simulink model "test0"  (R2016a)
settings: Solver=ode23  StartTime=0.0  StopTime=20  RelTol=1e-10
settings Model: Creator=wojta  LastModifiedBy=wojta

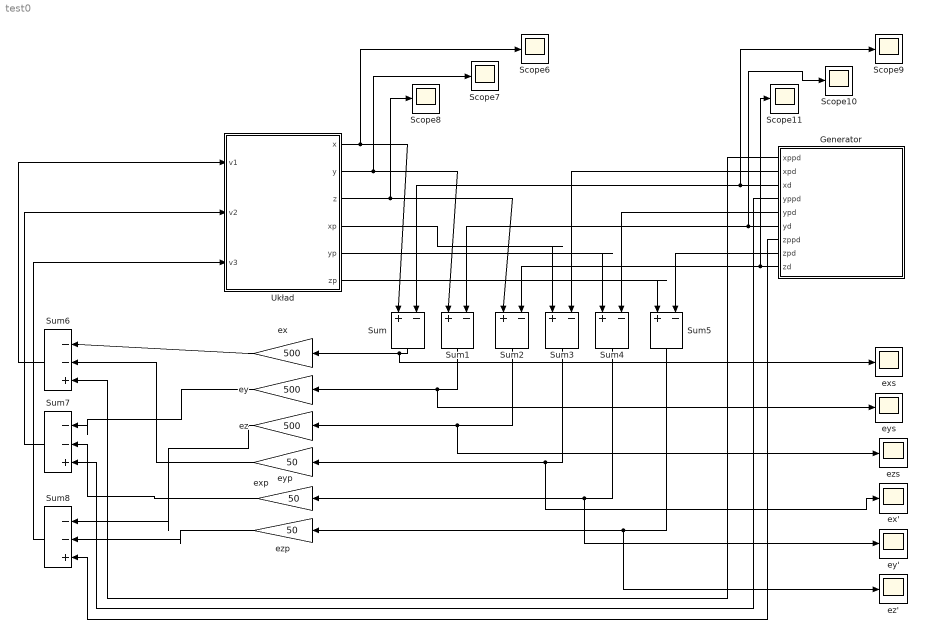
== system test0 ==
  Generator : Subsystem
  Scope{6..11} (6 alike) : Scope
  Sum{,1..5} (6 alike) : Sum  Inputs=|+-
  Sum6 : Sum  Inputs=|--+
  Sum7 : Sum  Inputs=|--+
  Sum8 : Sum  Inputs=|--+
  Układ : Subsystem
  ex : Gain  Gain=500
  ex' : Scope
  exp : Gain  Gain=50
  exs : Scope
  ey : Gain  Gain=500
  ey' : Scope
  eyp : Gain  Gain=50
  eys : Scope
  ez : Gain  Gain=500
  ez' : Scope
  ezp : Gain  Gain=50
  ezs : Scope
  wires:
  Układ/1(x) -> Scope6/1, Sum/1
  Generator/3(xd) -> Scope9/1, Sum/2
  Układ/2(y) -> Scope7/1, Sum1/1
  Generator/6(yd) -> Scope10/1, Sum1/2
  Układ/3(z) -> Scope8/1, Sum2/1
  Generator/9(zd) -> Scope11/1, Sum2/2
  Układ/4(xp) -> Sum3/1
  Generator/2(xpd) -> Sum3/2
  Układ/5(yp) -> Sum4/1
  Generator/5(ypd) -> Sum4/2
  Układ/6(zp) -> Sum5/1
  Generator/8(zpd) -> Sum5/2
  Sum/1 -> exs/1, ex/1
  Sum3/1 -> exp/1, ex'/1
  Sum4/1 -> ey'/1, eyp/1
  Sum5/1 -> ez'/1, ezp/1
  Sum2/1 -> ezs/1, ez/1
  Sum1/1 -> eys/1, ey/1
  ex/1 -> Sum6/1
  exp/1 -> Sum6/2
  Generator/1(xppd) -> Sum6/3
  Generator/4(yppd) -> Sum7/3
  Generator/7(zppd) -> Sum8/3
  ey/1 -> Sum7/1
  eyp/1 -> Sum7/2
  ezp/1 -> Sum8/2
  ez/1 -> Sum8/1
  Sum6/1 -> Układ/1(v1)
  Sum7/1 -> Układ/2(v2)
  Sum8/1 -> Układ/3(v3)

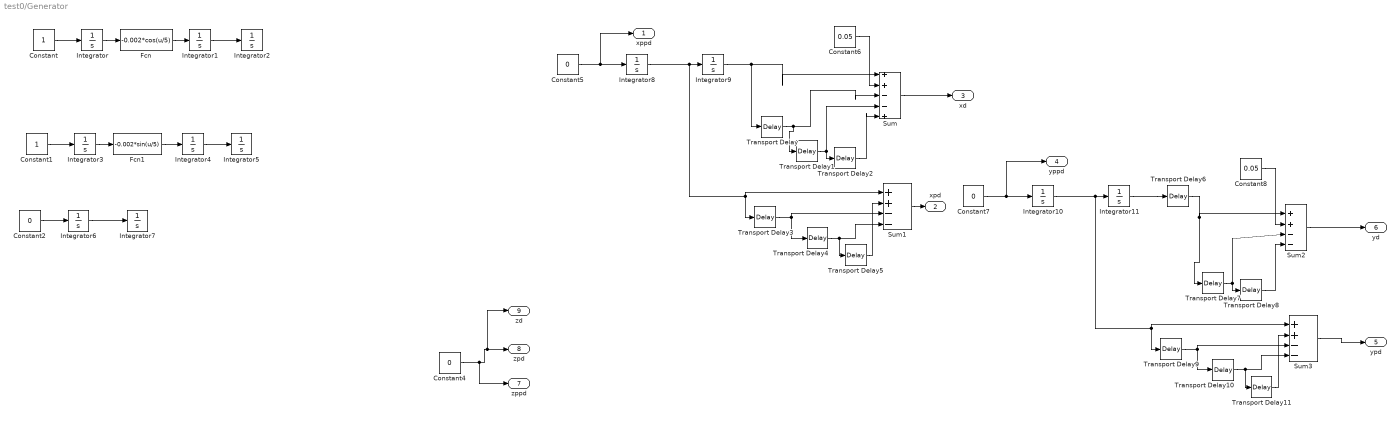
== system test0/Generator ==
  Constant : Constant
  Constant1 : Constant
  Constant{2,4..5,7} (4 alike) : Constant  Value=0
  Constant6 : Constant  Value=0.05
  Constant8 : Constant  Value=0.05
  Fcn : Fcn  Expr=-0.002*cos(u/5)
  Fcn1 : Fcn  Expr=-0.002*sin(u/5)
  Integrator{,1,3,5,7,9,11} (7 alike) : Integrator
  Integrator{4,6,8,10} (4 alike) : Integrator  InitialCondition=0.01
  Integrator2 : Integrator  InitialCondition=0.05
  Sum : Sum  Inputs=|++--+
  Sum1 : Sum  Inputs=|++--
  Sum2 : Sum  Inputs=|++--
  Sum3 : Sum  Inputs=|++--
  Transport Delay{,1..11} (12 alike) : TransportDelay  DelayTime=5
  xppd : Outport
  xpd : Outport  Port=2
  xd : Outport  Port=3
  yppd : Outport  Port=4
  ypd : Outport  Port=5
  yd : Outport  Port=6
  zppd : Outport  Port=7
  zpd : Outport  Port=8
  zd : Outport  Port=9
  wires:
  Constant/1 -> Integrator/1
  Integrator/1 -> Fcn/1
  Fcn/1 -> Integrator1/1
  Integrator1/1 -> Integrator2/1
  Constant1/1 -> Integrator3/1
  Integrator3/1 -> Fcn1/1
  Fcn1/1 -> Integrator4/1
  Integrator4/1 -> Integrator5/1
  Constant2/1 -> Integrator6/1
  Integrator6/1 -> Integrator7/1
  Constant4/1 -> zppd/1, zd/1, zpd/1
  Constant5/1 -> xppd/1, Integrator8/1
  Integrator8/1 -> Transport Delay3/1, Sum1/1, Integrator9/1
  Sum/1 -> xd/1
  Integrator9/1 -> Transport Delay/1, Sum/1
  Constant6/1 -> Sum/2
  Transport Delay/1 -> Transport Delay1/1, Sum/3
  Transport Delay1/1 -> Sum/4, Transport Delay2/1
  Transport Delay2/1 -> Sum/5
  Sum1/1 -> xpd/1
  Transport Delay3/1 -> Transport Delay4/1, Sum1/3
  Transport Delay4/1 -> Transport Delay5/1, Sum1/4
  Transport Delay5/1 -> Sum1/2
  Constant7/1 -> yppd/1, Integrator10/1
  Integrator10/1 -> Transport Delay9/1, Sum3/1, Integrator11/1
  Sum2/1 -> yd/1
  Integrator11/1 -> Transport Delay6/1
  Constant8/1 -> Sum2/2
  Transport Delay6/1 -> Sum2/1, Transport Delay7/1
  Transport Delay7/1 -> Sum2/3, Transport Delay8/1
  Transport Delay8/1 -> Sum2/4
  Transport Delay9/1 -> Transport Delay10/1, Sum3/3
  Transport Delay10/1 -> Transport Delay11/1, Sum3/4
  Transport Delay11/1 -> Sum3/2
  Sum3/1 -> ypd/1

== system test0/Układ ==
  v1 : Inport
  v2 : Inport  Port=2
  v3 : Inport  Port=3
  Constant3 : Constant  Value=1.6
  H : Subsystem
  O : Subsystem
  Obiekt : Subsystem
  Scope : Scope
  Scope1 : Scope
  Scope2 : Scope
  u : Subsystem
  x : Outport
  y : Outport  Port=2
  z : Outport  Port=3
  xp : Outport  Port=4
  yp : Outport  Port=5
  zp : Outport  Port=6
  wires:
  v3/1 -> u/3(v3)
  O/8(O32) -> u/14(O32)
  O/9(O33) -> u/15(O33)
  H/1(H1) -> u/4(H1)
  O/4(O21) -> u/10(O21)
  u/3(u3) -> Obiekt/3(u3)
  Obiekt/3(z) -> z/1, Scope2/1
  Obiekt/8(qp2) -> H/6(qp2)
  O/1(O11) -> u/7(O11)
  O/5(O22) -> u/11(O22)
  Obiekt/5(q2) -> H/3(q2), O/2(q2)
  Obiekt/7(qp3) -> H/7(qp3)
  H/3(H3) -> u/6(H3)
  H/2(H2) -> u/5(H2)
  Obiekt/4(q3) -> O/3(q3), H/4(q3)
  Obiekt/2(y) -> y/1, Scope1/1
  u/2(u2) -> Obiekt/2(u2)
  O/7(O31) -> u/13(O31)
  Obiekt/1(x) -> x/1, Scope/1
  Constant3/1 -> Obiekt/4(q4), O/4(q4), H/1(q4)
  Obiekt/9(qp1) -> H/5(qp1)
  O/2(O12) -> u/8(O12)
  u/1(u1) -> Obiekt/1(u1)
  O/3(O13) -> u/9(O13)
  Obiekt/6(q1) -> O/1(q1), H/2(q1)
  O/6(O23) -> u/12(O23)
  v1/1 -> u/1(v1)
  v2/1 -> u/2(v2)
  Obiekt/10(xp) -> xp/1
  Obiekt/11(yp) -> yp/1
  Obiekt/12(zp) -> zp/1

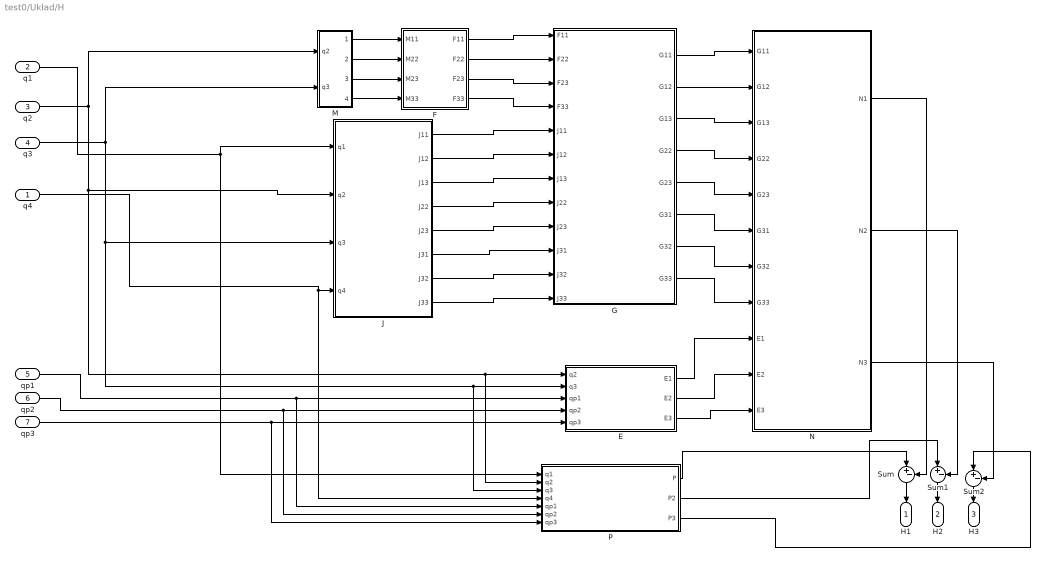
== system test0/Układ/H ==
  q4 : Inport
  q1 : Inport  Port=2
  q2 : Inport  Port=3
  q3 : Inport  Port=4
  qp1 : Inport  Port=5
  qp2 : Inport  Port=6
  qp3 : Inport  Port=7
  E : Subsystem
  F : Subsystem
  G : Subsystem
  J : Subsystem
  M : Subsystem
  N : Subsystem
  P : Subsystem
  Sum : Sum  Inputs=|+-
  Sum1 : Sum  Inputs=|+-
  Sum2 : Sum  Inputs=|+-
  H1 : Outport
  H2 : Outport  Port=2
  H3 : Outport  Port=3
  wires:
  q3/1 -> M/2(q3), P/3(q3), E/2(q3), J/3(q3)
  q1/1 -> P/1(q1), J/1(q1)
  q2/1 -> P/2(q2), E/1(q2), J/2(q2), M/1(q2)
  q4/1 -> P/4(q4), J/4(q4)
  F/1(F11) -> G/1(F11)
  F/2(F22) -> G/2(F22)
  F/3(F23) -> G/3(F23)
  F/4(F33) -> G/4(F33)
  J/1(J11) -> G/5(J11)
  J/2(J12) -> G/6(J12)
  J/3(J13) -> G/7(J13)
  J/4(J22) -> G/8(J22)
  J/5(J23) -> G/9(J23)
  J/6(J31) -> G/10(J31)
  J/7(J32) -> G/11(J32)
  J/8(J33) -> G/12(J33)
  qp1/1 -> P/5(qp1), E/3(qp1)
  qp2/1 -> P/6(qp2), E/4(qp2)
  qp3/1 -> P/7(qp3), E/5(qp3)
  E/3(E3) -> N/11(E3)
  E/2(E2) -> N/10(E2)
  E/1(E1) -> N/9(E1)
  G/8(G33) -> N/8(G33)
  G/7(G32) -> N/7(G32)
  G/6(G31) -> N/6(G31)
  G/5(G23) -> N/5(G23)
  G/4(G22) -> N/4(G22)
  G/2(G12) -> N/2(G12)
  G/3(G13) -> N/3(G13)
  G/1(G11) -> N/1(G11)
  Sum/1 -> H1/1
  Sum1/1 -> H2/1
  Sum2/1 -> H3/1
  N/1(N1) -> Sum/2
  N/2(N2) -> Sum1/2
  N/3(N3) -> Sum2/2
  P/1(P) -> Sum/1
  P/2(P2) -> Sum1/1
  P/3(P3) -> Sum2/1
  M/3(M23) -> F/3(M23)
  M/1(M11) -> F/1(M11)
  M/4("M33 ") -> F/4(M33)
  M/2(M22) -> F/2(M22)

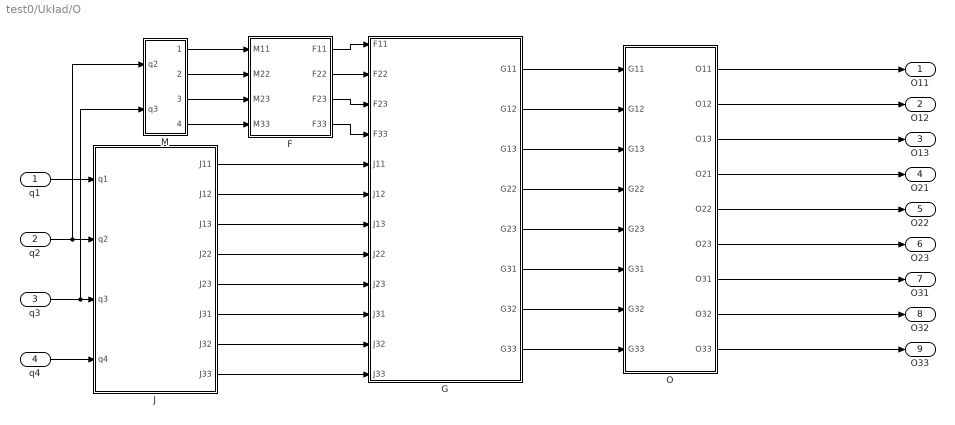
== system test0/Układ/O ==
  q1 : Inport
  q2 : Inport  Port=2
  q3 : Inport  Port=3
  q4 : Inport  Port=4
  F : Subsystem
  G : Subsystem
  J : Subsystem
  M : Subsystem
  O : Subsystem
  O11 : Outport
  O12 : Outport  Port=2
  O13 : Outport  Port=3
  O21 : Outport  Port=4
  O22 : Outport  Port=5
  O23 : Outport  Port=6
  O31 : Outport  Port=7
  O32 : Outport  Port=8
  O33 : Outport  Port=9
  wires:
  J/1(J11) -> G/5(J11)
  J/2(J12) -> G/6(J12)
  J/3(J13) -> G/7(J13)
  J/4(J22) -> G/8(J22)
  J/5(J23) -> G/9(J23)
  J/6(J31) -> G/10(J31)
  J/7(J32) -> G/11(J32)
  J/8(J33) -> G/12(J33)
  q3/1 -> J/3(q3), M/2(q3)
  q2/1 -> J/2(q2), M/1(q2)
  q1/1 -> J/1(q1)
  q4/1 -> J/4(q4)
  G/1(G11) -> O/1(G11)
  G/2(G12) -> O/2(G12)
  G/3(G13) -> O/3(G13)
  G/4(G22) -> O/4(G22)
  G/5(G23) -> O/5(G23)
  G/6(G31) -> O/6(G31)
  G/7(G32) -> O/7(G32)
  G/8(G33) -> O/8(G33)
  O/1(O11) -> O11/1
  O/2(O12) -> O12/1
  O/3(O13) -> O13/1
  O/4(O21) -> O21/1
  O/5(O22) -> O22/1
  O/6(O23) -> O23/1
  O/7(O31) -> O31/1
  O/8(O32) -> O32/1
  O/9(O33) -> O33/1
  M/3(M23) -> F/3(M23)
  M/1(M11) -> F/1(M11)
  M/4("M33 ") -> F/4(M33)
  M/2(M22) -> F/2(M22)
  F/1(F11) -> G/1(F11)
  F/2(F22) -> G/2(F22)
  F/3(F23) -> G/3(F23)
  F/4(F33) -> G/4(F33)

== system test0/Układ/Obiekt ==
  u1 : Inport
  u2 : Inport  Port=2
  u3 : Inport  Port=3
  q4 : Inport  Port=4
  Dynamika : Subsystem
  Kinematyka : Subsystem
  x : Outport
  y : Outport  Port=2
  z : Outport  Port=3
  q3 : Outport  Port=4
  q2 : Outport  Port=5
  q1 : Outport  Port=6
  qp3 : Outport  Port=7
  qp2 : Outport  Port=8
  qp1 : Outport  Port=9
  xp : Outport  Port=10
  yp : Outport  Port=11
  zp : Outport  Port=12
  wires:
  Dynamika/3(q3) -> q3/1, Kinematyka/3(q3)
  Dynamika/1(q1) -> q1/1, Kinematyka/1(q1)
  q4/1 -> Kinematyka/4(q4)
  Dynamika/2(q2) -> q2/1, Kinematyka/2(q2)
  Kinematyka/3(z) -> z/1
  Kinematyka/1(x) -> x/1
  Kinematyka/2(y) -> y/1
  u1/1 -> Dynamika/1(u1)
  u3/1 -> Dynamika/3(u3)
  u2/1 -> Dynamika/2(u2)
  Dynamika/4(qp3) -> Kinematyka/7(q3p), qp3/1
  Dynamika/6(qp1) -> Kinematyka/5(q1p), qp1/1
  Dynamika/5(qp2) -> Kinematyka/6(q2p), qp2/1
  Kinematyka/4(xp) -> xp/1
  Kinematyka/5(yp) -> yp/1
  Kinematyka/6(zp) -> zp/1

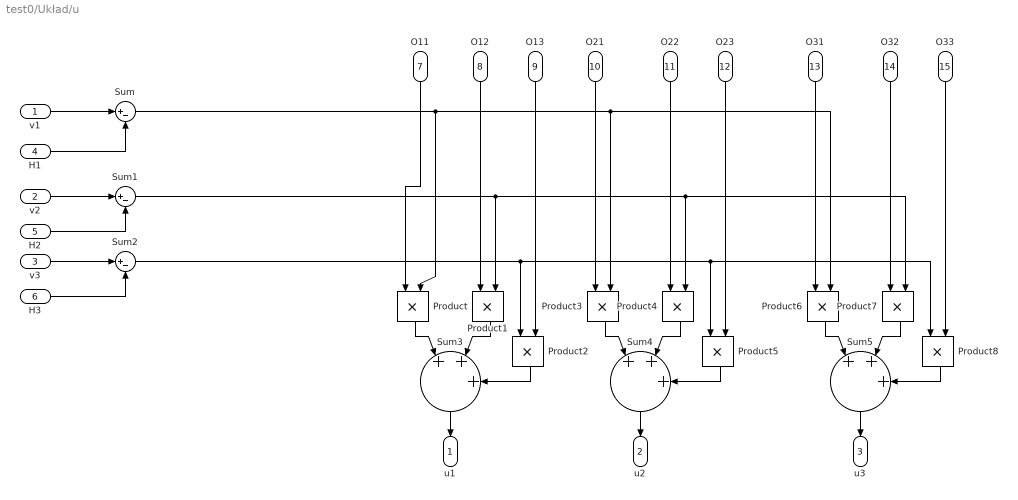
== system test0/Układ/u ==
  v1 : Inport
  v2 : Inport  Port=2
  v3 : Inport  Port=3
  H1 : Inport  Port=4
  H2 : Inport  Port=5
  H3 : Inport  Port=6
  O11 : Inport  Port=7
  O12 : Inport  Port=8
  O13 : Inport  Port=9
  O21 : Inport  Port=10
  O22 : Inport  Port=11
  O23 : Inport  Port=12
  O31 : Inport  Port=13
  O32 : Inport  Port=14
  O33 : Inport  Port=15
  Product{,1..8} (9 alike) : Product
  Sum : Sum  Inputs=|+-
  Sum1 : Sum  Inputs=|+-
  Sum2 : Sum  Inputs=|+-
  Sum3 : Sum  Inputs=|+++
  Sum4 : Sum  Inputs=|+++
  Sum5 : Sum  Inputs=|+++
  u1 : Outport
  u2 : Outport  Port=2
  u3 : Outport  Port=3
  wires:
  v1/1 -> Sum/1
  H1/1 -> Sum/2
  v2/1 -> Sum1/1
  H2/1 -> Sum1/2
  v3/1 -> Sum2/1
  H3/1 -> Sum2/2
  Sum3/1 -> u1/1
  Sum4/1 -> u2/1
  Sum5/1 -> u3/1
  Product/1 -> Sum3/1
  Product1/1 -> Sum3/2
  Product2/1 -> Sum3/3
  Product3/1 -> Sum4/1
  Product4/1 -> Sum4/2
  Product5/1 -> Sum4/3
  Product6/1 -> Sum5/1
  Product7/1 -> Sum5/2
  Product8/1 -> Sum5/3
  O11/1 -> Product/1
  Sum/1 -> Product/2, Product3/2, Product6/2
  Sum1/1 -> Product7/2, Product4/2, Product1/2
  Sum2/1 -> Product2/1, Product5/1, Product8/1
  O12/1 -> Product1/1
  O13/1 -> Product2/2
  O21/1 -> Product3/1
  O22/1 -> Product4/1
  O23/1 -> Product5/2
  O31/1 -> Product6/1
  O32/1 -> Product7/1
  O33/1 -> Product8/2

== system test0/Układ/H/E ==
  q2 : Inport
  q3 : Inport  Port=2
  qp1 : Inport  Port=3
  qp2 : Inport  Port=4
  qp3 : Inport  Port=5
  C : Subsystem
  D : Subsystem
  MATLAB Function : MATLAB Function  TreatAsAtomicUnit=on
  MATLAB Function1 : MATLAB Function  TreatAsAtomicUnit=on
  MATLAB Function2 : MATLAB Function  TreatAsAtomicUnit=on
  E1 : Outport
  E2 : Outport  Port=2
  E3 : Outport  Port=3
  wires:
  q3/1 -> D/2(q3), C/5(q3)
  qp1/1 -> C/1(qp1), MATLAB Function/1(qp1), MATLAB Function1/1(qp1), MATLAB Function2/1(qp1)
  qp2/1 -> C/2(qp2), MATLAB Function/2(qp2), MATLAB Function2/2(qp2)
  qp3/1 -> C/3(qp3), MATLAB Function/3(qp3), MATLAB Function1/2(qp3)
  q2/1 -> D/1(q2), C/4(q2)
  MATLAB Function/1(y) -> E1/1
  MATLAB Function1/1(y) -> E2/1
  MATLAB Function2/1(y) -> E3/1
  D/3(D3) -> MATLAB Function2/5(D3)
  C/5(C32) -> MATLAB Function2/4(C32)
  C/3(C13) -> MATLAB Function/6(C13), MATLAB Function2/3(C13)
  D/2(D2) -> MATLAB Function1/5(D2)
  C/4(C23) -> MATLAB Function1/4(C23)
  C/2(C12) -> MATLAB Function/5(C12), MATLAB Function1/3(C12)
  D/1(D1) -> MATLAB Function/7(D1)
  C/1(C11) -> MATLAB Function/4(C11)

== system test0/Układ/H/F ==
  M11 : Inport
  M22 : Inport  Port=2
  M23 : Inport  Port=3
  M33 : Inport  Port=4
  MATLAB Function : MATLAB Function  TreatAsAtomicUnit=on
  MATLAB Function1 : MATLAB Function  TreatAsAtomicUnit=on
  MATLAB Function2 : MATLAB Function  TreatAsAtomicUnit=on
  MATLAB Function3 : MATLAB Function  TreatAsAtomicUnit=on
  F11 : Outport
  F22 : Outport  Port=2
  F23 : Outport  Port=3
  F33 : Outport  Port=4
  wires:
  M11/1 -> MATLAB Function3/1(m11)
  MATLAB Function3/1(y) -> F11/1
  MATLAB Function/1(y) -> F22/1
  MATLAB Function1/1(y) -> F23/1
  MATLAB Function2/1(y) -> F33/1
  M22/1 -> MATLAB Function2/1(m22), MATLAB Function1/1(m22), MATLAB Function/1(m22)
  M23/1 -> MATLAB Function2/2(m23), MATLAB Function1/2(m23), MATLAB Function/2(m23)
  M33/1 -> MATLAB Function2/3(m33), MATLAB Function1/3(m33), MATLAB Function/3(m33)

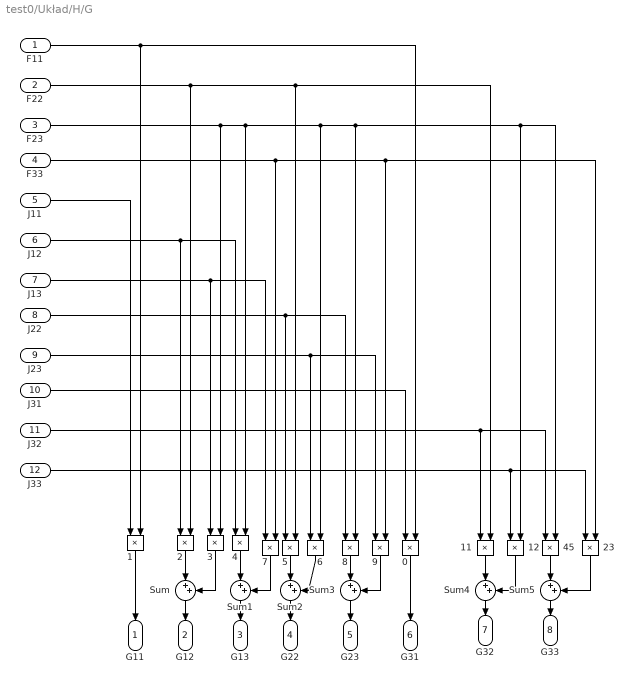
== system test0/Układ/H/G ==
  F11 : Inport
  F22 : Inport  Port=2
  F23 : Inport  Port=3
  F33 : Inport  Port=4
  J11 : Inport  Port=5
  J12 : Inport  Port=6
  J13 : Inport  Port=7
  J22 : Inport  Port=8
  J23 : Inport  Port=9
  J31 : Inport  Port=10
  J32 : Inport  Port=11
  J33 : Inport  Port=12
  {0..9,11..12,23,45} (14 alike) : Product
  Sum{,1..5} (6 alike) : Sum  Inputs=|++
  G11 : Outport
  G12 : Outport  Port=2
  G13 : Outport  Port=3
  G22 : Outport  Port=4
  G23 : Outport  Port=5
  G31 : Outport  Port=6
  G32 : Outport  Port=7
  G33 : Outport  Port=8
  wires:
  Sum5/1 -> G33/1
  Sum4/1 -> G32/1
  Sum3/1 -> G23/1
  Sum2/1 -> G22/1
  Sum1/1 -> G13/1
  Sum/1 -> G12/1
  1/1 -> G11/1
  2/1 -> Sum/1
  3/1 -> Sum/2
  4/1 -> Sum1/1
  7/1 -> Sum1/2
  5/1 -> Sum2/1
  6/1 -> Sum2/2
  8/1 -> Sum3/1
  9/1 -> Sum3/2
  0/1 -> G31/1
  11/1 -> Sum4/1
  12/1 -> Sum4/2
  45/1 -> Sum5/1
  23/1 -> Sum5/2
  F33/1 -> 7/2, 9/2, 23/2
  J33/1 -> 12/1, 23/1
  F23/1 -> 3/2, 4/2, 6/2, 8/2, 12/2, 45/2
  J32/1 -> 11/1, 45/1
  F22/1 -> 5/2, 11/2, 2/2
  F11/1 -> 0/2, 1/2
  J31/1 -> 0/1
  J23/1 -> 6/1, 9/1
  J22/1 -> 5/1, 8/1
  J13/1 -> 3/1, 7/1
  J12/1 -> 2/1, 4/1
  J11/1 -> 1/1

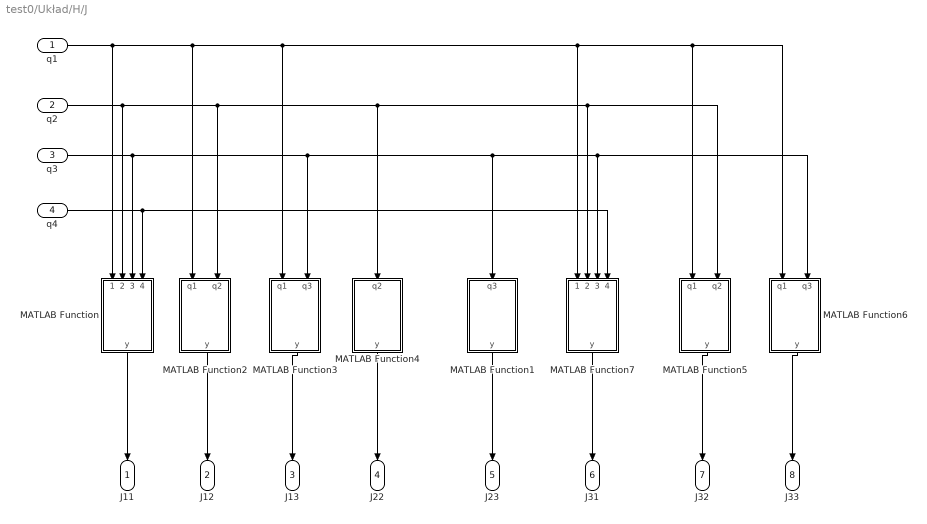
== system test0/Układ/H/J ==
  q1 : Inport
  q2 : Inport  Port=2
  q3 : Inport  Port=3
  q4 : Inport  Port=4
  MATLAB Function : MATLAB Function  TreatAsAtomicUnit=on
  MATLAB Function1 : MATLAB Function  TreatAsAtomicUnit=on
  MATLAB Function2 : MATLAB Function  TreatAsAtomicUnit=on
  MATLAB Function3 : MATLAB Function  TreatAsAtomicUnit=on
  MATLAB Function4 : MATLAB Function  TreatAsAtomicUnit=on
  MATLAB Function5 : MATLAB Function  TreatAsAtomicUnit=on
  MATLAB Function6 : MATLAB Function  TreatAsAtomicUnit=on
  MATLAB Function7 : MATLAB Function  TreatAsAtomicUnit=on
  J11 : Outport
  J12 : Outport  Port=2
  J13 : Outport  Port=3
  J22 : Outport  Port=4
  J23 : Outport  Port=5
  J31 : Outport  Port=6
  J32 : Outport  Port=7
  J33 : Outport  Port=8
  wires:
  MATLAB Function/1(y) -> J11/1
  MATLAB Function2/1(y) -> J12/1
  MATLAB Function3/1(y) -> J13/1
  MATLAB Function4/1(y) -> J22/1
  MATLAB Function1/1(y) -> J23/1
  MATLAB Function7/1(y) -> J31/1
  MATLAB Function5/1(y) -> J32/1
  MATLAB Function6/1(y) -> J33/1
  q4/1 -> MATLAB Function7/4(q4), MATLAB Function/4(q4)
  q3/1 -> MATLAB Function/3(q3), MATLAB Function3/2(q3), MATLAB Function1/1(q3), MATLAB Function7/3(q3), MATLAB Function6/2(q3)
  q2/1 -> MATLAB Function/2(q2), MATLAB Function2/2(q2), MATLAB Function7/2(q2), MATLAB Function5/2(q2), MATLAB Function4/1(q2)
  q1/1 -> MATLAB Function/1(q1), MATLAB Function2/1(q1), MATLAB Function3/1(q1), MATLAB Function7/1(q1), MATLAB Function5/1(q1), MATLAB Function6/1(q1)

== system test0/Układ/H/M ==
  q2 : Inport
  q3 : Inport  Port=2
  Constant : Constant  Value=6.56125
  Constant1 : Constant  Value=4.624
  Constant2 : Constant  Value=10.9
  Constant3 : Constant  Value=4.624
  MATLAB Function : MATLAB Function  TreatAsAtomicUnit=on
  MATLAB Function1 : MATLAB Function  TreatAsAtomicUnit=on
  Sum : Sum  Inputs=|++
  Sum1 : Sum  Inputs=|++
  M11 : Outport
  M22 : Outport  Port=2
  M23 : Outport  Port=3
  "M33 " : Outport  Port=4
  wires:
  MATLAB Function/1(y) -> M11/1
  q2/1 -> MATLAB Function1/1(q2), MATLAB Function/1(q2)
  q3/1 -> MATLAB Function1/2(q3), MATLAB Function/2(q3)
  Sum/1 -> M22/1
  Constant/1 -> Sum/1
  Constant1/1 -> Sum/2
  Constant2/1 -> Sum1/1
  Constant3/1 -> Sum1/2
  Sum1/1 -> "M33 "/1
  MATLAB Function1/1(y) -> M23/1

== system test0/Układ/H/N ==
  G11 : Inport
  G12 : Inport  Port=2
  G13 : Inport  Port=3
  G22 : Inport  Port=4
  G23 : Inport  Port=5
  G31 : Inport  Port=6
  G32 : Inport  Port=7
  G33 : Inport  Port=8
  E1 : Inport  Port=9
  E2 : Inport  Port=10
  E3 : Inport  Port=11
  Constant : Constant  Value=0
  MATLAB Function : MATLAB Function  TreatAsAtomicUnit=on
  MATLAB Function1 : MATLAB Function  TreatAsAtomicUnit=on
  MATLAB Function2 : MATLAB Function  TreatAsAtomicUnit=on
  N1 : Outport
  N2 : Outport  Port=2
  N3 : Outport  Port=3
  wires:
  MATLAB Function/1(y) -> N1/1
  MATLAB Function1/1(y) -> N2/1
  MATLAB Function2/1(y) -> N3/1
  E3/1 -> MATLAB Function/6(E3), MATLAB Function1/6(E3), MATLAB Function2/6(E3)
  E2/1 -> MATLAB Function/5(E2), MATLAB Function1/5(E2), MATLAB Function2/5(E2)
  E1/1 -> MATLAB Function/4(E1), MATLAB Function2/4(E1), MATLAB Function1/4(E1)
  G11/1 -> MATLAB Function/1(G11)
  G12/1 -> MATLAB Function/2(G12)
  G13/1 -> MATLAB Function/3(G13)
  G22/1 -> MATLAB Function1/2(G22)
  Constant/1 -> MATLAB Function1/1(G21)
  G23/1 -> MATLAB Function1/3(G23)
  G31/1 -> MATLAB Function2/1(G31)
  G32/1 -> MATLAB Function2/2(G32)
  G33/1 -> MATLAB Function2/3(G33)

== system test0/Układ/H/P ==
  q1 : Inport
  q2 : Inport  Port=2
  q3 : Inport  Port=3
  q4 : Inport  Port=4
  qp1 : Inport  Port=5
  qp2 : Inport  Port=6
  qp3 : Inport  Port=7
  MATLAB Function : MATLAB Function  TreatAsAtomicUnit=on
  MATLAB Function1 : MATLAB Function  TreatAsAtomicUnit=on
  MATLAB Function2 : MATLAB Function  TreatAsAtomicUnit=on
  P : Outport
  P2 : Outport  Port=2
  P3 : Outport  Port=3
  wires:
  MATLAB Function/1(y) -> P/1
  MATLAB Function2/1(y) -> P2/1
  MATLAB Function1/1(y) -> P3/1
  qp3/1 -> MATLAB Function/7(qp3), MATLAB Function2/5(qp3), MATLAB Function1/7(qp3)
  qp1/1 -> MATLAB Function/5(qp1), MATLAB Function2/3(qp1), MATLAB Function1/5(qp1)
  q4/1 -> MATLAB Function1/4(q4), MATLAB Function/4(q4)
  q3/1 -> MATLAB Function/3(q3), MATLAB Function2/2(q3), MATLAB Function1/3(q3)
  q2/1 -> MATLAB Function/2(q2), MATLAB Function1/2(q2), MATLAB Function2/1(q2)
  q1/1 -> MATLAB Function1/1(q1), MATLAB Function/1(q1)
  qp2/1 -> MATLAB Function/6(qp2), MATLAB Function2/4(qp2), MATLAB Function1/6(qp2)

== system test0/Układ/O/F ==
  M11 : Inport
  M22 : Inport  Port=2
  M23 : Inport  Port=3
  M33 : Inport  Port=4
  MATLAB Function : MATLAB Function  TreatAsAtomicUnit=on
  MATLAB Function1 : MATLAB Function  TreatAsAtomicUnit=on
  MATLAB Function2 : MATLAB Function  TreatAsAtomicUnit=on
  MATLAB Function3 : MATLAB Function  TreatAsAtomicUnit=on
  F11 : Outport
  F22 : Outport  Port=2
  F23 : Outport  Port=3
  F33 : Outport  Port=4
  wires:
  M11/1 -> MATLAB Function3/1(m11)
  MATLAB Function3/1(y) -> F11/1
  MATLAB Function/1(y) -> F22/1
  MATLAB Function1/1(y) -> F23/1
  MATLAB Function2/1(y) -> F33/1
  M22/1 -> MATLAB Function2/1(m22), MATLAB Function1/1(m22), MATLAB Function/1(m22)
  M23/1 -> MATLAB Function2/2(m23), MATLAB Function1/2(m23), MATLAB Function/2(m23)
  M33/1 -> MATLAB Function2/3(m33), MATLAB Function1/3(m33), MATLAB Function/3(m33)

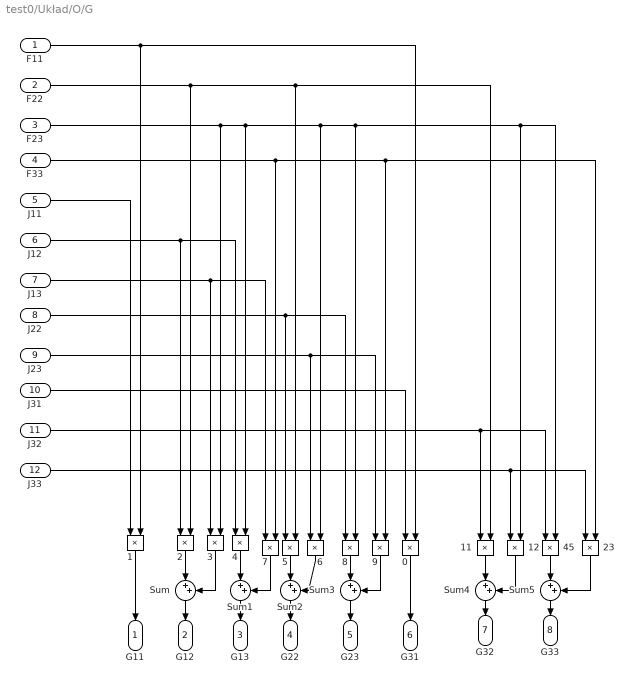
== system test0/Układ/O/G ==
  F11 : Inport
  F22 : Inport  Port=2
  F23 : Inport  Port=3
  F33 : Inport  Port=4
  J11 : Inport  Port=5
  J12 : Inport  Port=6
  J13 : Inport  Port=7
  J22 : Inport  Port=8
  J23 : Inport  Port=9
  J31 : Inport  Port=10
  J32 : Inport  Port=11
  J33 : Inport  Port=12
  {0..9,11..12,23,45} (14 alike) : Product
  Sum{,1..5} (6 alike) : Sum  Inputs=|++
  G11 : Outport
  G12 : Outport  Port=2
  G13 : Outport  Port=3
  G22 : Outport  Port=4
  G23 : Outport  Port=5
  G31 : Outport  Port=6
  G32 : Outport  Port=7
  G33 : Outport  Port=8
  wires:
  Sum5/1 -> G33/1
  Sum4/1 -> G32/1
  Sum3/1 -> G23/1
  Sum2/1 -> G22/1
  Sum1/1 -> G13/1
  Sum/1 -> G12/1
  1/1 -> G11/1
  2/1 -> Sum/1
  3/1 -> Sum/2
  4/1 -> Sum1/1
  7/1 -> Sum1/2
  5/1 -> Sum2/1
  6/1 -> Sum2/2
  8/1 -> Sum3/1
  9/1 -> Sum3/2
  0/1 -> G31/1
  11/1 -> Sum4/1
  12/1 -> Sum4/2
  45/1 -> Sum5/1
  23/1 -> Sum5/2
  F33/1 -> 7/2, 9/2, 23/2
  J33/1 -> 12/1, 23/1
  F23/1 -> 3/2, 4/2, 6/2, 8/2, 12/2, 45/2
  J32/1 -> 11/1, 45/1
  F22/1 -> 5/2, 11/2, 2/2
  F11/1 -> 0/2, 1/2
  J31/1 -> 0/1
  J23/1 -> 6/1, 9/1
  J22/1 -> 5/1, 8/1
  J13/1 -> 3/1, 7/1
  J12/1 -> 2/1, 4/1
  J11/1 -> 1/1

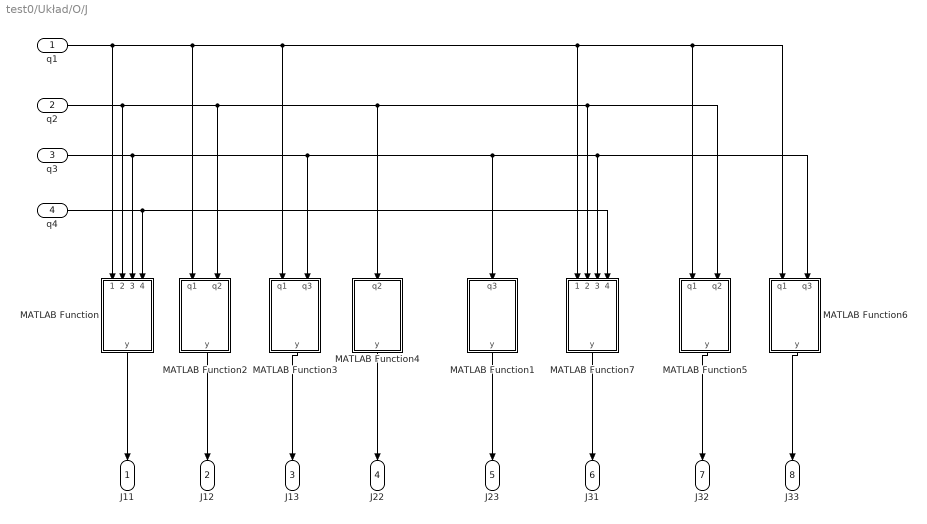
== system test0/Układ/O/J ==
  q1 : Inport
  q2 : Inport  Port=2
  q3 : Inport  Port=3
  q4 : Inport  Port=4
  MATLAB Function : MATLAB Function  TreatAsAtomicUnit=on
  MATLAB Function1 : MATLAB Function  TreatAsAtomicUnit=on
  MATLAB Function2 : MATLAB Function  TreatAsAtomicUnit=on
  MATLAB Function3 : MATLAB Function  TreatAsAtomicUnit=on
  MATLAB Function4 : MATLAB Function  TreatAsAtomicUnit=on
  MATLAB Function5 : MATLAB Function  TreatAsAtomicUnit=on
  MATLAB Function6 : MATLAB Function  TreatAsAtomicUnit=on
  MATLAB Function7 : MATLAB Function  TreatAsAtomicUnit=on
  J11 : Outport
  J12 : Outport  Port=2
  J13 : Outport  Port=3
  J22 : Outport  Port=4
  J23 : Outport  Port=5
  J31 : Outport  Port=6
  J32 : Outport  Port=7
  J33 : Outport  Port=8
  wires:
  MATLAB Function/1(y) -> J11/1
  MATLAB Function2/1(y) -> J12/1
  MATLAB Function3/1(y) -> J13/1
  MATLAB Function4/1(y) -> J22/1
  MATLAB Function1/1(y) -> J23/1
  MATLAB Function7/1(y) -> J31/1
  MATLAB Function5/1(y) -> J32/1
  MATLAB Function6/1(y) -> J33/1
  q4/1 -> MATLAB Function7/4(q4), MATLAB Function/4(q4)
  q3/1 -> MATLAB Function/3(q3), MATLAB Function3/2(q3), MATLAB Function1/1(q3), MATLAB Function7/3(q3), MATLAB Function6/2(q3)
  q2/1 -> MATLAB Function/2(q2), MATLAB Function2/2(q2), MATLAB Function7/2(q2), MATLAB Function5/2(q2), MATLAB Function4/1(q2)
  q1/1 -> MATLAB Function/1(q1), MATLAB Function2/1(q1), MATLAB Function3/1(q1), MATLAB Function7/1(q1), MATLAB Function5/1(q1), MATLAB Function6/1(q1)

== system test0/Układ/O/M ==
  q2 : Inport
  q3 : Inport  Port=2
  Constant : Constant  Value=6.56125
  Constant1 : Constant  Value=4.624
  Constant2 : Constant  Value=10.9
  Constant3 : Constant  Value=4.624
  MATLAB Function : MATLAB Function  TreatAsAtomicUnit=on
  MATLAB Function1 : MATLAB Function  TreatAsAtomicUnit=on
  Sum : Sum  Inputs=|++
  Sum1 : Sum  Inputs=|++
  M11 : Outport
  M22 : Outport  Port=2
  M23 : Outport  Port=3
  "M33 " : Outport  Port=4
  wires:
  MATLAB Function/1(y) -> M11/1
  q2/1 -> MATLAB Function1/1(q2), MATLAB Function/1(q2)
  q3/1 -> MATLAB Function1/2(q3), MATLAB Function/2(q3)
  Sum/1 -> M22/1
  Constant/1 -> Sum/1
  Constant1/1 -> Sum/2
  Constant2/1 -> Sum1/1
  Constant3/1 -> Sum1/2
  Sum1/1 -> "M33 "/1
  MATLAB Function1/1(y) -> M23/1

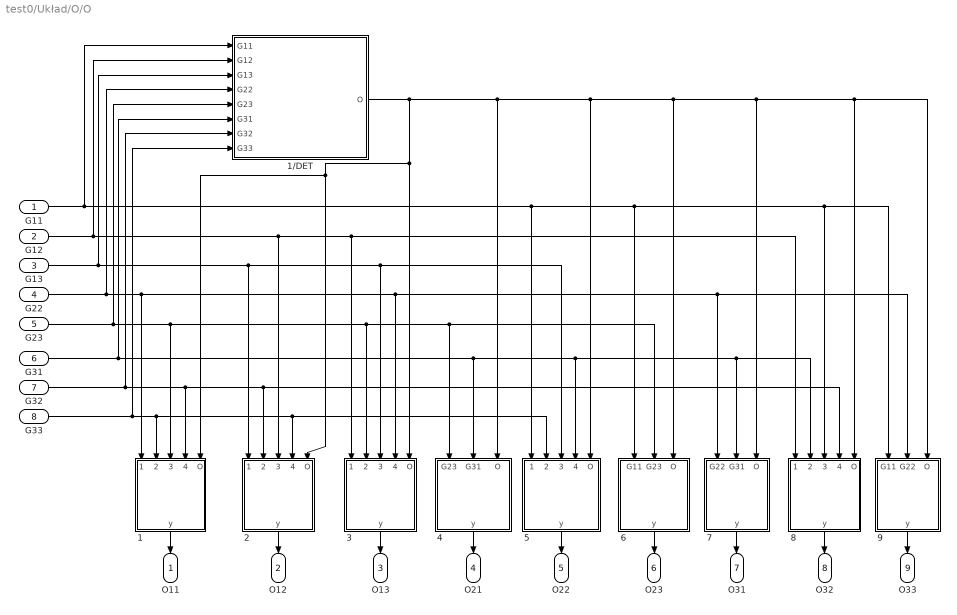
== system test0/Układ/O/O ==
  G11 : Inport
  G12 : Inport  Port=2
  G13 : Inport  Port=3
  G22 : Inport  Port=4
  G23 : Inport  Port=5
  G31 : Inport  Port=6
  G32 : Inport  Port=7
  G33 : Inport  Port=8
  1 : MATLAB Function  TreatAsAtomicUnit=on
  1/DET : MATLAB Function  TreatAsAtomicUnit=on
  2 : MATLAB Function  TreatAsAtomicUnit=on
  3 : MATLAB Function  TreatAsAtomicUnit=on
  4 : MATLAB Function  TreatAsAtomicUnit=on
  5 : MATLAB Function  TreatAsAtomicUnit=on
  6 : MATLAB Function  TreatAsAtomicUnit=on
  7 : MATLAB Function  TreatAsAtomicUnit=on
  8 : MATLAB Function  TreatAsAtomicUnit=on
  9 : MATLAB Function  TreatAsAtomicUnit=on
  O11 : Outport
  O12 : Outport  Port=2
  O13 : Outport  Port=3
  O21 : Outport  Port=4
  O22 : Outport  Port=5
  O23 : Outport  Port=6
  O31 : Outport  Port=7
  O32 : Outport  Port=8
  O33 : Outport  Port=9
  wires:
  1/1(y) -> O11/1
  2/1(y) -> O12/1
  3/1(y) -> O13/1
  4/1(y) -> O21/1
  5/1(y) -> O22/1
  6/1(y) -> O23/1
  7/1(y) -> O31/1
  8/1(y) -> O32/1
  9/1(y) -> O33/1
  1/DET/1(O) -> 4/3(O), 5/5(O), 6/3(O), 7/3(O), 8/5(O), 9/3(O), 1/5(O), 2/5(O), 3/5(O)
  G22/1 -> 1/DET/4(G22), 1/1(G22), 3/4(G22), 7/1(G22), 9/2(G22)
  G11/1 -> 1/DET/1(G11), 5/1(G11), 6/1(G11), 8/3(G11), 9/1(G11)
  G31/1 -> 1/DET/6(G31), 4/2(G31), 5/4(G31), 7/2(G31), 8/2(G31)
  G12/1 -> 1/DET/2(G12), 8/1(G12), 3/1(G12), 2/3(G12)
  G23/1 -> 1/DET/5(G23), 3/2(G23), 4/1(G23), 6/2(G23), 1/3(G23)
  G13/1 -> 1/DET/3(G13), 2/1(G13), 3/3(G13), 5/3(G13)
  G33/1 -> 1/DET/8(G33), 1/2(G33), 2/4(G33), 5/2(G33)
  G32/1 -> 1/DET/7(G32), 1/4(G32), 2/2(G32), 8/4(G32)

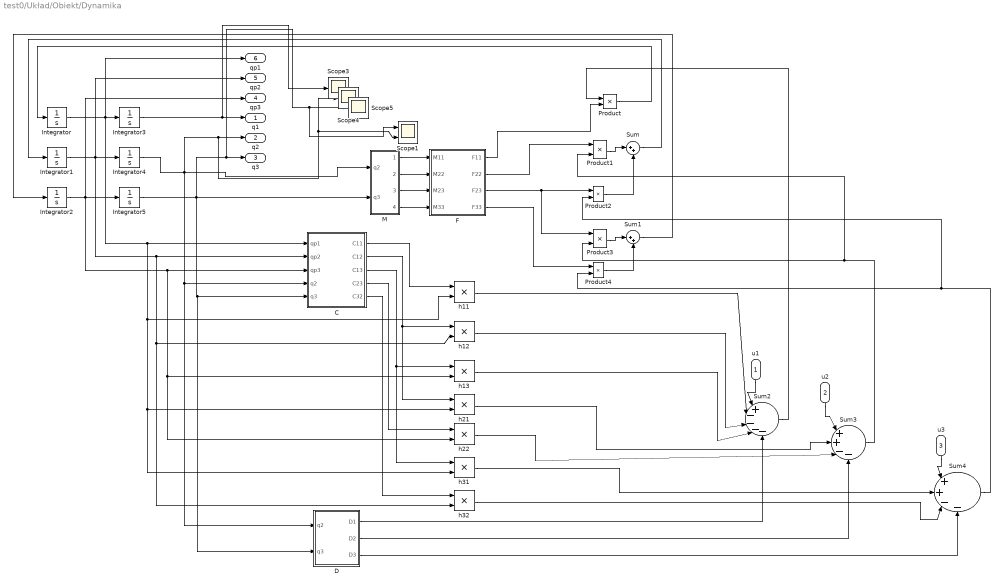
== system test0/Układ/Obiekt/Dynamika ==
  u1 : Inport
  u2 : Inport  Port=2
  u3 : Inport  Port=3
  C : Subsystem
  D : Subsystem
  F : Subsystem
  Integrator : Integrator
  Integrator1 : Integrator
  Integrator2 : Integrator
  Integrator3 : Integrator  InitialCondition=1
  Integrator4 : Integrator  InitialCondition=0.4
  Integrator5 : Integrator  InitialCondition=0.1
  M : Subsystem
  Product{,1..4} (5 alike) : Product
  Scope1 : Scope  NumInputPorts=2
  Scope3 : Scope
  Scope4 : Scope
  Scope5 : Scope
  Sum : Sum  Inputs=|++
  Sum1 : Sum  Inputs=|++
  Sum2 : Sum  Inputs=|+----
  Sum3 : Sum  Inputs=|++--
  Sum4 : Sum  Inputs=|++--
  h{11..13,21..22,31..32} (7 alike) : Product
  q1 : Outport
  q2 : Outport  Port=2
  q3 : Outport  Port=3
  qp3 : Outport  Port=4
  qp2 : Outport  Port=5
  qp1 : Outport  Port=6
  wires:
  Sum1/1 -> Integrator2/1
  Integrator/1 -> qp1/1, h31/2, h21/2, h11/2, C/1(qp1), Integrator3/1
  Integrator1/1 -> qp2/1, h32/2, h12/2, C/2(qp2), Integrator4/1
  Product/1 -> Integrator/1
  Integrator2/1 -> qp3/1, h22/2, h13/2, C/3(qp3), Integrator5/1
  Integrator4/1 -> D/1(q2), C/4(q2), M/1(q2), Scope4/1, Scope1/2, q2/1
  Integrator5/1 -> Scope1/1, Scope5/1, q3/1, D/2(q3), C/5(q3), M/2(q3)
  Sum/1 -> Integrator1/1
  M/3(M23) -> F/3(M23)
  Sum2/1 -> Product/1
  Integrator3/1 -> Scope3/1, q1/1
  Product3/1 -> Sum1/1
  h12/1 -> Sum2/3
  Sum3/1 -> Product1/2, Product3/2
  Sum4/1 -> Product2/2, Product4/2
  Product1/1 -> Sum/1
  D/2(D2) -> Sum3/4
  M/1(M11) -> F/1(M11)
  D/3(D3) -> Sum4/4
  C/1(C11) -> h11/1
  F/3(F23) -> Product3/1, Product2/1
  F/4(F33) -> Product4/1
  C/3(C13) -> h31/1, h13/1
  h11/1 -> Sum2/2
  Product4/1 -> Sum1/2
  D/1(D1) -> Sum2/5
  C/4(C23) -> h22/1
  C/5(C32) -> h32/1
  h21/1 -> Sum3/2
  h22/1 -> Sum3/3
  M/4("M33 ") -> F/4(M33)
  M/2(M22) -> F/2(M22)
  Product2/1 -> Sum/2
  F/2(F22) -> Product1/1
  h13/1 -> Sum2/4
  C/2(C12) -> h21/1, h12/1
  F/1(F11) -> Product/2
  u2/1 -> Sum3/1
  h31/1 -> Sum4/2
  h32/1 -> Sum4/3
  u3/1 -> Sum4/1
  u1/1 -> Sum2/1

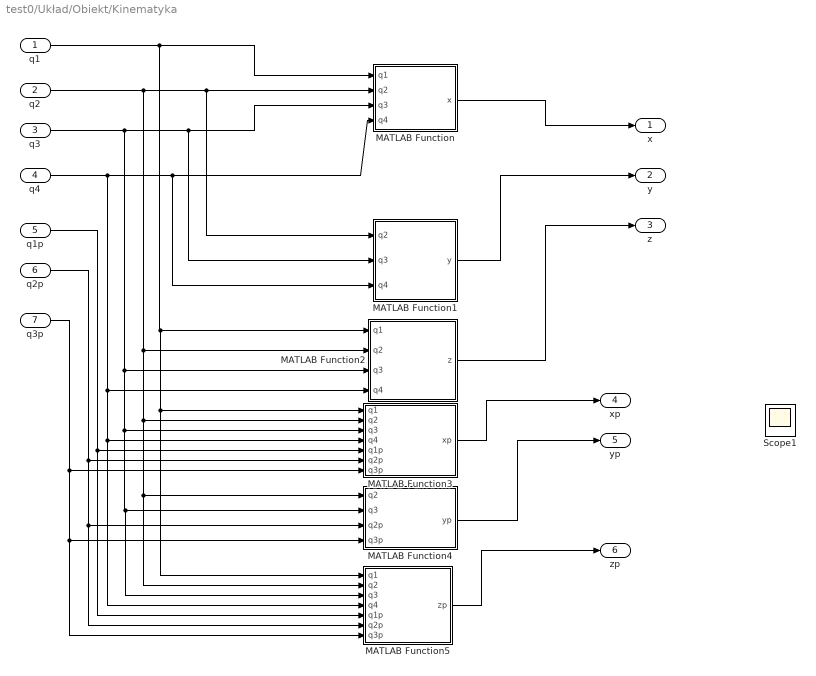
== system test0/Układ/Obiekt/Kinematyka ==
  q1 : Inport
  q2 : Inport  Port=2
  q3 : Inport  Port=3
  q4 : Inport  Port=4
  q1p : Inport  Port=5
  q2p : Inport  Port=6
  q3p : Inport  Port=7
  MATLAB Function : MATLAB Function  TreatAsAtomicUnit=on
  MATLAB Function1 : MATLAB Function  TreatAsAtomicUnit=on
  MATLAB Function2 : MATLAB Function  TreatAsAtomicUnit=on
  MATLAB Function3 : MATLAB Function  TreatAsAtomicUnit=on
  MATLAB Function4 : MATLAB Function  TreatAsAtomicUnit=on
  MATLAB Function5 : MATLAB Function  TreatAsAtomicUnit=on
  Scope1 : Scope
  x : Outport
  y : Outport  Port=2
  z : Outport  Port=3
  xp : Outport  Port=4
  yp : Outport  Port=5
  zp : Outport  Port=6
  wires:
  MATLAB Function/1(x) -> x/1
  MATLAB Function2/1(z) -> z/1
  q1/1 -> MATLAB Function5/1(q1), MATLAB Function3/1(q1), MATLAB Function2/1(q1), MATLAB Function/1(q1)
  q2/1 -> MATLAB Function5/2(q2), MATLAB Function4/1(q2), MATLAB Function3/2(q2), MATLAB Function2/2(q2), MATLAB Function1/1(q2), MATLAB Function/2(q2)
  q3/1 -> MATLAB Function5/3(q3), MATLAB Function4/2(q3), MATLAB Function3/3(q3), MATLAB Function2/3(q3), MATLAB Function1/2(q3), MATLAB Function/3(q3)
  q4/1 -> MATLAB Function5/4(q4), MATLAB Function3/4(q4), MATLAB Function2/4(q4), MATLAB Function1/3(q4), MATLAB Function/4(q4)
  MATLAB Function3/1(xp) -> xp/1
  MATLAB Function4/1(yp) -> yp/1
  MATLAB Function5/1(zp) -> zp/1
  q1p/1 -> MATLAB Function5/5(q1p), MATLAB Function3/5(q1p)
  q2p/1 -> MATLAB Function5/6(q2p), MATLAB Function4/3(q2p), MATLAB Function3/6(q2p)
  q3p/1 -> MATLAB Function5/7(q3p), MATLAB Function4/4(q3p), MATLAB Function3/7(q3p)
  MATLAB Function1/1(y) -> y/1

== system test0/Układ/H/E/C ==
  qp1 : Inport
  qp2 : Inport  Port=2
  qp3 : Inport  Port=3
  q2 : Inport  Port=4
  q3 : Inport  Port=5
  MATLAB Function : MATLAB Function  TreatAsAtomicUnit=on
  MATLAB Function1 : MATLAB Function  TreatAsAtomicUnit=on
  MATLAB Function2 : MATLAB Function  TreatAsAtomicUnit=on
  MATLAB Function3 : MATLAB Function  TreatAsAtomicUnit=on
  MATLAB Function4 : MATLAB Function  TreatAsAtomicUnit=on
  C11 : Outport
  C12 : Outport  Port=2
  C13 : Outport  Port=3
  C23 : Outport  Port=4
  C32 : Outport  Port=5
  wires:
  MATLAB Function/1(y) -> C11/1
  MATLAB Function1/1(y) -> C12/1
  MATLAB Function2/1(y) -> C13/1
  MATLAB Function3/1(y) -> C23/1
  MATLAB Function4/1(y) -> C32/1
  qp1/1 -> MATLAB Function2/1(qp1), MATLAB Function1/1(qp1)
  qp2/1 -> MATLAB Function/1(qp2), MATLAB Function4/1(qp2), MATLAB Function3/1(qp2)
  q2/1 -> MATLAB Function/3(q2), MATLAB Function1/2(q2), MATLAB Function2/2(q2), MATLAB Function4/2(q2), MATLAB Function3/3(q2)
  q3/1 -> MATLAB Function/4(q3), MATLAB Function1/3(q3), MATLAB Function2/3(q3), MATLAB Function4/3(q3), MATLAB Function3/4(q3)
  qp3/1 -> MATLAB Function3/2(qp3), MATLAB Function/2(qp3)

== system test0/Układ/H/E/D ==
  q2 : Inport
  q3 : Inport  Port=2
  Constant : Constant  Value=0
  MATLAB Function : MATLAB Function  TreatAsAtomicUnit=on
  MATLAB Function1 : MATLAB Function  TreatAsAtomicUnit=on
  D1 : Outport
  D2 : Outport  Port=2
  D3 : Outport  Port=3
  wires:
  Constant/1 -> D1/1
  MATLAB Function1/1(y) -> D3/1
  MATLAB Function/1(y) -> D2/1
  q2/1 -> MATLAB Function/1(q2)
  q3/1 -> MATLAB Function1/1(q3)

== system test0/Układ/Obiekt/Dynamika/C ==
  qp1 : Inport
  qp2 : Inport  Port=2
  qp3 : Inport  Port=3
  q2 : Inport  Port=4
  q3 : Inport  Port=5
  MATLAB Function : MATLAB Function  TreatAsAtomicUnit=on
  MATLAB Function1 : MATLAB Function  TreatAsAtomicUnit=on
  MATLAB Function2 : MATLAB Function  TreatAsAtomicUnit=on
  MATLAB Function3 : MATLAB Function  TreatAsAtomicUnit=on
  MATLAB Function4 : MATLAB Function  TreatAsAtomicUnit=on
  C11 : Outport
  C12 : Outport  Port=2
  C13 : Outport  Port=3
  C23 : Outport  Port=4
  C32 : Outport  Port=5
  wires:
  MATLAB Function/1(y) -> C11/1
  MATLAB Function1/1(y) -> C12/1
  MATLAB Function2/1(y) -> C13/1
  MATLAB Function3/1(y) -> C23/1
  MATLAB Function4/1(y) -> C32/1
  qp1/1 -> MATLAB Function2/1(qp1), MATLAB Function1/1(qp1)
  qp2/1 -> MATLAB Function/1(qp2), MATLAB Function4/1(qp2), MATLAB Function3/1(qp2)
  q2/1 -> MATLAB Function/3(q2), MATLAB Function1/2(q2), MATLAB Function2/2(q2), MATLAB Function4/2(q2), MATLAB Function3/3(q2)
  q3/1 -> MATLAB Function/4(q3), MATLAB Function1/3(q3), MATLAB Function2/3(q3), MATLAB Function4/3(q3), MATLAB Function3/4(q3)
  qp3/1 -> MATLAB Function3/2(qp3), MATLAB Function/2(qp3)

== system test0/Układ/Obiekt/Dynamika/D ==
  q2 : Inport
  q3 : Inport  Port=2
  Constant : Constant  Value=0
  MATLAB Function : MATLAB Function  TreatAsAtomicUnit=on
  MATLAB Function1 : MATLAB Function  TreatAsAtomicUnit=on
  D1 : Outport
  D2 : Outport  Port=2
  D3 : Outport  Port=3
  wires:
  Constant/1 -> D1/1
  MATLAB Function1/1(y) -> D3/1
  MATLAB Function/1(y) -> D2/1
  q2/1 -> MATLAB Function/1(q2)
  q3/1 -> MATLAB Function1/1(q3)

== system test0/Układ/Obiekt/Dynamika/F ==
  M11 : Inport
  M22 : Inport  Port=2
  M23 : Inport  Port=3
  M33 : Inport  Port=4
  MATLAB Function : MATLAB Function  TreatAsAtomicUnit=on
  MATLAB Function1 : MATLAB Function  TreatAsAtomicUnit=on
  MATLAB Function2 : MATLAB Function  TreatAsAtomicUnit=on
  MATLAB Function3 : MATLAB Function  TreatAsAtomicUnit=on
  F11 : Outport
  F22 : Outport  Port=2
  F23 : Outport  Port=3
  F33 : Outport  Port=4
  wires:
  M11/1 -> MATLAB Function3/1(m11)
  MATLAB Function3/1(y) -> F11/1
  MATLAB Function/1(y) -> F22/1
  MATLAB Function1/1(y) -> F23/1
  MATLAB Function2/1(y) -> F33/1
  M22/1 -> MATLAB Function2/1(m22), MATLAB Function1/1(m22), MATLAB Function/1(m22)
  M23/1 -> MATLAB Function2/2(m23), MATLAB Function1/2(m23), MATLAB Function/2(m23)
  M33/1 -> MATLAB Function2/3(m33), MATLAB Function1/3(m33), MATLAB Function/3(m33)

== system test0/Układ/Obiekt/Dynamika/M ==
  q2 : Inport
  q3 : Inport  Port=2
  Constant : Constant  Value=6.56125
  Constant1 : Constant  Value=4.624
  Constant2 : Constant  Value=10.9
  Constant3 : Constant  Value=4.624
  MATLAB Function : MATLAB Function  TreatAsAtomicUnit=on
  MATLAB Function1 : MATLAB Function  TreatAsAtomicUnit=on
  Sum : Sum  Inputs=|++
  Sum1 : Sum  Inputs=|++
  M11 : Outport
  M22 : Outport  Port=2
  M23 : Outport  Port=3
  "M33 " : Outport  Port=4
  wires:
  MATLAB Function/1(y) -> M11/1
  q2/1 -> MATLAB Function1/1(q2), MATLAB Function/1(q2)
  q3/1 -> MATLAB Function1/2(q3), MATLAB Function/2(q3)
  Sum/1 -> M22/1
  Constant/1 -> Sum/1
  Constant1/1 -> Sum/2
  Constant2/1 -> Sum1/1
  Constant3/1 -> Sum1/2
  Sum1/1 -> "M33 "/1
  MATLAB Function1/1(y) -> M23/1

== matlab function test0/Układ/Obiekt/Dynamika/M/MATLAB Function1 ==
  data: q2 input; y output; q3 input
function y = fcn(q2, q3)
%#codegen

y=-0.25*-0.531*sin(q2+q3);

== matlab function test0/Układ/Obiekt/Dynamika/M/MATLAB Function ==
  data: q2 input; y output; q3 input
function y = fcn(q2, q3)
%#codegen

y=5.66+6.56125*(sin(q2))^2+-0.531*sin(q2)*cos(q3)+10.9*(cos(q3))^2;

== matlab function test0/Układ/Obiekt/Dynamika/F/MATLAB Function ==
  data: m22 input; y output; m23 input; m33 input
function y = fcn(m22, m23, m33)
%#codegen

y = m33/(m22*m33-(m23*m23));

== matlab function test0/Układ/Obiekt/Dynamika/F/MATLAB Function1 ==
  data: m22 input; y output; m23 input; m33 input
function y = fcn(m22, m23, m33)
%#codegen

y = -m23/(m22*m33-(m23*m23));

== matlab function test0/Układ/Obiekt/Dynamika/F/MATLAB Function2 ==
  data: m22 input; y output; m23 input; m33 input
function y = fcn(m22, m23, m33)
%#codegen

y = m22/(m22*m33-(m23*m23));

== matlab function test0/Układ/Obiekt/Dynamika/F/MATLAB Function3 ==
  data: m11 input; y output
function y = fcn(m11)
%#codegen

y = (m11)^(-1);

== matlab function test0/Układ/Obiekt/Dynamika/C/MATLAB Function ==
  data: qp2 input; y output; qp3 input; q2 input; q3 input
function y = fcn(qp2, qp3, q2, q3)
%#codegen

y = qp2*0.5*(6.56125*sin(2*q2)-0.531*cos(q2)*cos(q3))-qp3*0.5*(-0.531*sin(q2)*sin(q3)+10.9*sin(2*q3));

== matlab function test0/Układ/Obiekt/Dynamika/C/MATLAB Function1 ==
  data: qp1 input; y output; q2 input; q3 input
function y = fcn(qp1, q2, q3)
%#codegen

y = 0.5*qp1*(6.56125*sin(2*q2)-0.531*cos(q2)*cos(q3));

== matlab function test0/Układ/Obiekt/Dynamika/C/MATLAB Function2 ==
  data: qp1 input; y output; q2 input; q3 input
function y = fcn(qp1, q2, q3)
%#codegen

y = -0.5*qp1*(-0.531*sin(q2)*sin(q3)+10.9*sin(2*q3));

== matlab function test0/Układ/Obiekt/Dynamika/C/MATLAB Function3 ==
  data: qp2 input; y output; qp3 input; q2 input; q3 input
function y = fcn(qp2, qp3, q2, q3)
%#codegen

y = -0.5*(qp2+0.5*qp3)*(-0.531*cos(q2+q3));

== matlab function test0/Układ/Obiekt/Dynamika/C/MATLAB Function4 ==
  data: qp2 input; y output; q2 input; q3 input
function y = fcn(qp2, q2, q3)
%#codegen

y = 0.25*qp2*(-0.531)*cos(q2+q3);

== matlab function test0/Układ/Obiekt/Dynamika/D/MATLAB Function ==
  data: q2 input; y output
function y = fcn(q2)
%#codegen

y = -145*sin(q2);

== matlab function test0/Układ/Obiekt/Dynamika/D/MATLAB Function1 ==
  data: q3 input; y output
function y = fcn(q3)
%#codegen

y = -5.7879*cos(q3);

== matlab function test0/Układ/Obiekt/Kinematyka/MATLAB Function ==
  data: q1 input; x output; q2 input; q3 input; q4 input
function x = fcn(q1, q2, q3, q4)
%#codegen

x = cos(q1)*(0.45*cos(q2)+0.67*cos(q3)+0.095*sin(q4));

== matlab function test0/Układ/Obiekt/Kinematyka/MATLAB Function1 ==
  data: q2 input; y output; q3 input; q4 input
function y = fcn(q2, q3, q4)
%#codegen

y = 0.095*cos(q4)-0.45*sin(q2)-0.67*sin(q3)-0.7;

== matlab function test0/Układ/Obiekt/Kinematyka/MATLAB Function2 ==
  data: q1 input; z output; q2 input; q3 input; q4 input
function z = fcn(q1, q2, q3, q4)
%#codegen

z = sin(q1)*(0.45*cos(q2)+0.67*cos(q3)+0.095*sin(q4));

== matlab function test0/Układ/H/F/MATLAB Function ==
  data: m22 input; y output; m23 input; m33 input
function y = fcn(m22, m23, m33)
%#codegen

y = m33/(m22*m33-(m23*m23));

== matlab function test0/Układ/H/F/MATLAB Function1 ==
  data: m22 input; y output; m23 input; m33 input
function y = fcn(m22, m23, m33)
%#codegen

y = -m23/(m22*m33-(m23*m23));

== matlab function test0/Układ/H/F/MATLAB Function2 ==
  data: m22 input; y output; m23 input; m33 input
function y = fcn(m22, m23, m33)
%#codegen

y = m22/(m22*m33-(m23*m23));

== matlab function test0/Układ/H/F/MATLAB Function3 ==
  data: m11 input; y output
function y = fcn(m11)
%#codegen

y = (m11)^(-1);

== matlab function test0/Układ/H/M/MATLAB Function ==
  data: q2 input; y output; q3 input
function y = fcn(q2, q3)
%#codegen

y=5.66+6.56125*(sin(q2))^2+-0.531*sin(q2)*cos(q3)+10.9*(cos(q3))^2;

== matlab function test0/Układ/H/M/MATLAB Function1 ==
  data: q2 input; y output; q3 input
function y = fcn(q2, q3)
%#codegen

y=-0.25*-0.531*sin(q2+q3);

== matlab function test0/Układ/H/J/MATLAB Function ==
  data: q1 input; y output; q2 input; q3 input; q4 input
function y = fcn(q1, q2, q3, q4)
%#codegen

y = -sin(q1)*(0.45*cos(q2)+0.67*cos(q3)+0.095*sin(q4));

== matlab function test0/Układ/H/J/MATLAB Function1 ==
  data: q3 input; y output
function y = fcn(q3)
%#codegen

y = -0.67*cos(q3);

== matlab function test0/Układ/H/J/MATLAB Function2 ==
  data: q1 input; y output; q2 input
function y = fcn(q1, q2)
%#codegen

y = -0.45*cos(q1)*sin(q2);

== matlab function test0/Układ/H/J/MATLAB Function3 ==
  data: q1 input; y output; q3 input
function y = fcn(q1,q3)
%#codegen

y = -0.67*cos(q1)*sin(q3);

== matlab function test0/Układ/H/J/MATLAB Function4 ==
  data: q2 input; y output
function y = fcn(q2)
%#codegen

y = -0.45*cos(q2);

== matlab function test0/Układ/H/J/MATLAB Function5 ==
  data: q1 input; y output; q2 input
function y = fcn(q1, q2)
%#codegen

y = -0.45*sin(q1)*sin(q2);

== matlab function test0/Układ/H/J/MATLAB Function6 ==
  data: q1 input; y output; q3 input
function y = fcn(q1, q3)
%#codegen

y = -0.67*sin(q1)*sin(q3);

== matlab function test0/Układ/H/J/MATLAB Function7 ==
  data: q1 input; y output; q2 input; q3 input; q4 input
function y = fcn(q1, q2, q3, q4)
%#codegen

y = cos(q1)*(0.45*cos(q2)+0.67*cos(q3)+0.095*sin(q4));

== matlab function test0/Układ/O/F/MATLAB Function ==
  data: m22 input; y output; m23 input; m33 input
function y = fcn(m22, m23, m33)
%#codegen

y = m33/(m22*m33-(m23*m23));

== matlab function test0/Układ/O/F/MATLAB Function1 ==
  data: m22 input; y output; m23 input; m33 input
function y = fcn(m22, m23, m33)
%#codegen

y = -m23/(m22*m33-(m23*m23));

== matlab function test0/Układ/O/F/MATLAB Function2 ==
  data: m22 input; y output; m23 input; m33 input
function y = fcn(m22, m23, m33)
%#codegen

y = m22/(m22*m33-(m23*m23));

== matlab function test0/Układ/O/F/MATLAB Function3 ==
  data: m11 input; y output
function y = fcn(m11)
%#codegen

y = (m11)^(-1);

== matlab function test0/Układ/O/M/MATLAB Function ==
  data: q2 input; y output; q3 input
function y = fcn(q2, q3)
%#codegen

y=5.66+6.56125*(sin(q2))^2+-0.531*sin(q2)*cos(q3)+10.9*(cos(q3))^2;

== matlab function test0/Układ/O/M/MATLAB Function1 ==
  data: q2 input; y output; q3 input
function y = fcn(q2, q3)
%#codegen

y=-0.25*-0.531*sin(q2+q3);

== matlab function test0/Układ/O/J/MATLAB Function ==
  data: q1 input; y output; q2 input; q3 input; q4 input
function y = fcn(q1, q2, q3, q4)
%#codegen

y = -sin(q1)*(0.45*cos(q2)+0.67*cos(q3)+0.095*sin(q4));

== matlab function test0/Układ/H/E/MATLAB Function ==
  data: qp1 input; y output; qp2 input; qp3 input; C11 input; C12 input; C13 input; D1 input
function y = fcn(qp1,qp2,qp3,C11,C12,C13,D1)
%#codegen

y = C11*qp1+C12*qp2+C13*qp3+D1;

== matlab function test0/Układ/H/E/MATLAB Function1 ==
  data: qp1 input; y output; qp3 input; C12 input; C23 input; D2 input
function y = fcn(qp1, qp3,C12,C23,D2)
%#codegen

y = -C12*qp1+C23*qp3+D2;

== matlab function test0/Układ/H/E/MATLAB Function2 ==
  data: qp1 input; y output; qp2 input; C13 input; C32 input; D3 input
function y = fcn(qp1,qp2,C13,C32,D3)
%#codegen

y = -C13*qp1+C32*qp2+D3;

== matlab function test0/Układ/H/N/MATLAB Function ==
  data: G11 input; y output; G12 input; G13 input; E1 input; E2 input; E3 input
function y = fcn(G11,G12,G13,E1,E2,E3)
%#codegen

y = G11*E1+G12*E2+G13*E3;

== matlab function test0/Układ/H/N/MATLAB Function1 ==
  data: G21 input; y output; G22 input; G23 input; E1 input; E2 input; E3 input
function y = fcn(G21,G22,G23,E1,E2,E3)
%#codegen

y = G21*E1+G22*E2+G23*E3;

== matlab function test0/Układ/H/N/MATLAB Function2 ==
  data: G31 input; y output; G32 input; G33 input; E1 input; E2 input; E3 input
function y = fcn(G31,G32,G33,E1,E2,E3)
%#codegen

y = G31*E1+G32*E2+G33*E3;

== matlab function test0/Układ/H/P/MATLAB Function ==
  data: q1 input; y output; q2 input; q3 input; q4 input; qp1 input; qp2 input; qp3 input
function y = fcn(q1,q2,q3,q4,qp1,qp2,qp3)
%#codegen

y = qp1*(-qp1*cos(q1)*(0.45*cos(q2)+0.67*cos(q3)+0.095*sin(q4))+qp2*0.45*sin(q1)*sin(q2)-qp3*0.67*sin(q1)*sin(q3))+qp2*(-qp1*sin(q1)*(-0.45*sin(q2)+0.67*cos(q3)+0.095*sin(q4))-qp2*0.45*cos(q1)*cos(q2))+qp3*(-qp1*sin(q1)*(0.45*cos(q2)-0.67*sin(q3)+0.095*sin(q4))-qp3*cos(q1)*cos(q3));

== matlab function test0/Układ/O/J/MATLAB Function1 ==
  data: q3 input; y output
function y = fcn(q3)
%#codegen

y = -0.67*cos(q3);

== matlab function test0/Układ/O/J/MATLAB Function2 ==
  data: q1 input; y output; q2 input
function y = fcn(q1, q2)
%#codegen

y = -0.45*cos(q1)*sin(q2);

== matlab function test0/Układ/O/J/MATLAB Function3 ==
  data: q1 input; y output; q3 input
function y = fcn(q1,q3)
%#codegen

y = -0.67*cos(q1)*sin(q3);

== matlab function test0/Układ/O/J/MATLAB Function4 ==
  data: q2 input; y output
function y = fcn(q2)
%#codegen

y = -0.45*cos(q2);

== matlab function test0/Układ/O/J/MATLAB Function5 ==
  data: q1 input; y output; q2 input
function y = fcn(q1, q2)
%#codegen

y = -0.45*sin(q1)*sin(q2);

== matlab function test0/Układ/O/J/MATLAB Function6 ==
  data: q1 input; y output; q3 input
function y = fcn(q1, q3)
%#codegen

y = -0.67*sin(q1)*sin(q3);

== matlab function test0/Układ/O/J/MATLAB Function7 ==
  data: q1 input; y output; q2 input; q3 input; q4 input
function y = fcn(q1, q2, q3, q4)
%#codegen

y = cos(q1)*(0.45*cos(q2)+0.67*cos(q3)+0.095*sin(q4));

== matlab function test0/Układ/Obiekt/Kinematyka/MATLAB Function3 ==
  data: q1 input; xp output; q2 input; q3 input; q4 input; q1p input; q2p input; q3p input
function xp = fcn(q1, q2, q3, q4, q1p, q2p, q3p)
%#codegen

xp = -q1p*sin(q1)*0.45*cos(q2)-q2p*cos(q1)*0.45*sin(q2)-q1p*sin(q1)*0.67*cos(q3)-q3p*cos(q1)*0.67*sin(q3)-q1p*sin(q1)*0.095*sin(q4);

== matlab function test0/Układ/Obiekt/Kinematyka/MATLAB Function4 ==
  data: q2 input; yp output; q3 input; q2p input; q3p input
function yp = fcn( q2, q3, q2p, q3p)
%#codegen

yp =-0.45*cos(q2)*q2p-0.67*cos(q3)*q3p;

== matlab function test0/Układ/Obiekt/Kinematyka/MATLAB Function5 ==
  data: q1 input; zp output; q2 input; q3 input; q4 input; q1p input; q2p input; q3p input
function zp = fcn(q1, q2, q3, q4, q1p, q2p, q3p)
%#codegen

zp = q1p*cos(q1)*0.45*cos(q2)-q2p*sin(q1)*0.45*sin(q2)+q1p*cos(q1)*0.67*cos(q3)-q3p*sin(q1)*0.67*sin(q3)+q1p*cos(q1)*0.095*sin(q4);

== matlab function test0/Układ/O/O/1 ==
  data: G22 input; y output; G33 input; G23 input; G32 input; O input
function y = fcn(G22,G33,G23,G32,O)
%#codegen

y = O*(G22*G33-G23*G32);

== matlab function test0/Układ/O/O/2 ==
  data: G13 input; y output; G32 input; G12 input; G33 input; O input
function y = fcn(G13,G32,G12,G33,O)
%#codegen

y = O*(G13*G32-G12*G33);

== matlab function test0/Układ/O/O/3 ==
  data: G12 input; y output; G23 input; G13 input; G22 input; O input
function y = fcn(G12,G23,G13,G22,O)
%#codegen

y = O*(G12*G23-G13*G22);

== matlab function test0/Układ/O/O/4 ==
  data: G23 input; y output; G31 input; O input
function y = fcn(G23,G31,O)
%#codegen

y = O*(G23*G31);

== matlab function test0/Układ/O/O/5 ==
  data: G11 input; y output; G33 input; G13 input; G31 input; O input
function y = fcn(G11,G33,G13,G31,O)
%#codegen

y = O*(G11*G33-G13*G31);

== matlab function test0/Układ/O/O/6 ==
  data: G11 input; y output; G23 input; O input
function y = fcn(G11,G23,O)
%#codegen

y = O*(-G11*G23);

== matlab function test0/Układ/O/O/7 ==
  data: G22 input; y output; G31 input; O input
function y = fcn(G22,G31,O)
%#codegen

y = O*(-G22*G31);

== matlab function test0/Układ/O/O/8 ==
  data: G12 input; y output; G31 input; G11 input; G32 input; O input
function y = fcn(G12,G31,G11,G32,O)
%#codegen

y = O*(G12*G31-G11*G32);

== matlab function test0/Układ/O/O/9 ==
  data: G11 input; y output; G22 input; O input
function y = fcn(G11,G22,O)
%#codegen

y = O*(G22*G11);

== matlab function test0/Układ/O/O/1//DET ==
  data: G11 input; O output; G12 input; G13 input; G22 input; G23 input; G31 input; G32 input; G33 input
function O = fcn(G11,G12,G13,G22,G23,G31,G32,G33)
%#codegen

O = 1/(G11*G22*G33+G31*G12*G23-G11*G32*G23-G31*G22*G13);

== matlab function test0/Układ/H/P/MATLAB Function1 ==
  data: q1 input; y output; q2 input; q3 input; q4 input; qp1 input; qp2 input; qp3 input
function y = fcn(q1,q2,q3,q4,qp1,qp2,qp3)
%#codegen

y = qp1*(-qp1*sin(q1)*(0.45*cos(q2)+0.67*cos(q3)+0.095*sin(q4))-qp2*0.45*cos(q1)*sin(q2)-qp3*0.67*cos(q1)*sin(q3))+qp2*(-qp1*0.45*cos(q1)*sin(q2)-qp2*0.45*sin(q1)*cos(q2))+qp3*(-qp1*0.67*cos(q1)*sin(q3)-qp3*0.67*sin(q1)*cos(q3));

== matlab function test0/Układ/H/P/MATLAB Function2 ==
  data: y output; q2 input; q3 input; qp1 input; qp2 input; qp3 input
function y = fcn(q2,q3,qp1,qp2,qp3)
%#codegen

y = qp1*0+qp2*(qp2*0.45*sin(q2))+qp3*qp3*0.67*sin(q3);

== matlab function test0/Układ/H/E/C/MATLAB Function ==
  data: qp2 input; y output; qp3 input; q2 input; q3 input
function y = fcn(qp2, qp3, q2, q3)
%#codegen

y = qp2*0.5*(6.56125*sin(2*q2)-0.531*cos(q2)*cos(q3))-qp3*0.5*(-0.531*sin(q2)*sin(q3)+10.9*sin(2*q3));

== matlab function test0/Układ/H/E/C/MATLAB Function1 ==
  data: qp1 input; y output; q2 input; q3 input
function y = fcn(qp1, q2, q3)
%#codegen

y = 0.5*qp1*(6.56125*sin(2*q2)-0.531*cos(q2)*cos(q3));

== matlab function test0/Układ/H/E/C/MATLAB Function2 ==
  data: qp1 input; y output; q2 input; q3 input
function y = fcn(qp1, q2, q3)
%#codegen

y = -0.5*qp1*(-0.531*sin(q2)*sin(q3)+10.9*sin(2*q3));

== matlab function test0/Układ/H/E/C/MATLAB Function3 ==
  data: qp2 input; y output; qp3 input; q2 input; q3 input
function y = fcn(qp2, qp3, q2, q3)
%#codegen

y = -0.5*(qp2+0.5*qp3)*(-0.531*cos(q2+q3));

== matlab function test0/Układ/H/E/C/MATLAB Function4 ==
  data: qp2 input; y output; q2 input; q3 input
function y = fcn(qp2, q2, q3)
%#codegen

y = 0.25*qp2*(-0.531)*cos(q2+q3);

== matlab function test0/Układ/H/E/D/MATLAB Function ==
  data: q2 input; y output
function y = fcn(q2)
%#codegen

y = -145*sin(q2);

== matlab function test0/Układ/H/E/D/MATLAB Function1 ==
  data: q3 input; y output
function y = fcn(q3)
%#codegen

y = -5.7879*cos(q3);
